simulink model "flexpes_phctrlr_backup_jun3_2022"  (R2020a)
settings: Solver=VariableStepAuto  StartTime=0.0  StopTime=10.0  RelTol=1e-3
undefined symbols (not defined in the file): debouncer_cycles, F_lock_thr, FPGA_CLK, FPGA_Ts, IIR_C_X, IIR_C_X1, IIR_C_Y1, max_unwrap_periods, PFD_CLK, PFD_Ts, PH_lock_thr, PHCTRLR_CLK, PHCTRLR_Ts, TDC_cnt_per_period, unwrap_res_period_thr, unwrap_res_thr, wrap_detect_thr
libraries: xbsIndex_r4 x277
(part 2 of 2)

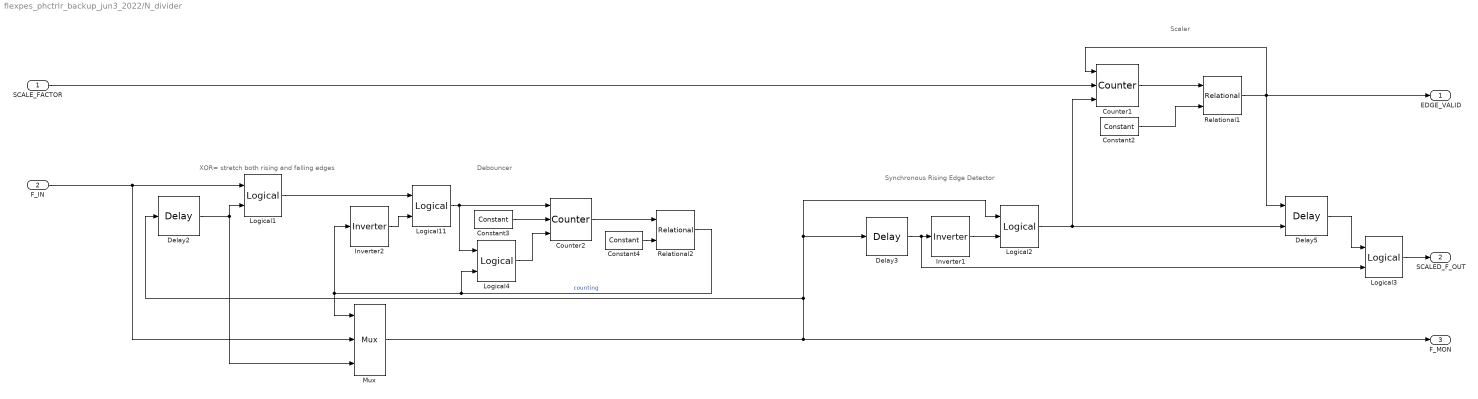
== system flexpes_phctrlr_backup_jun3_2022/N_divider ==
  note: XOR= stretch both rising and falling edges
  note: Debouncer
  note: Scaler
  note: Synchronous Rising Edge Detector
  SCALE_FACTOR : Inport
  F_IN : Inport  Port=2
  Constant2 : xbsIndex_r4/Constant  const=1.0  gui_display_data_type=Fixed-point  arith_type=Unsigned  n_bits=10  bin_pt=0  preci_type=Single  exp_width=8  frac_width=24  explicit_period=off  period=1  equ=P=C  opselect=C  inp2=PCIN>>17  opr=+  inp1=P  carry=CIN  dbl_ovrd=off  block_type=constant
  Constant3 : xbsIndex_r4/Constant  const=debouncer_cycles  gui_display_data_type=Fixed-point  arith_type=Unsigned  n_bits=7  bin_pt=0  preci_type=Single  exp_width=8  frac_width=24  explicit_period=off  period=1  equ=P=C  opselect=C  inp2=PCIN>>17  opr=+  inp1=P  carry=CIN  dbl_ovrd=off  block_type=constant
  Constant4 : xbsIndex_r4/Constant  const=1  gui_display_data_type=Fixed-point  arith_type=Unsigned  n_bits=7  bin_pt=0  preci_type=Single  exp_width=8  frac_width=24  explicit_period=off  period=1  equ=P=C  opselect=C  inp2=PCIN>>17  opr=+  inp1=P  carry=CIN  dbl_ovrd=off  block_type=constant
  Counter1 : xbsIndex_r4/Counter  cnt_type=Free Running  cnt_to=2  operation=Down  start_count=1  cnt_by_val=1  arith_type=Unsigned  n_bits=10  bin_pt=0  load_pin=on  rst=off  en=on  explicit_period=on  period=FPGA_Ts  use_behavioral_HDL=off  implementation=Fabric  dbl_ovrd=off  block_type=counter
  Counter2 : xbsIndex_r4/Counter  cnt_type=Free Running  cnt_to=2  operation=Down  start_count=1  cnt_by_val=1  arith_type=Unsigned  n_bits=7  bin_pt=0  load_pin=on  rst=off  en=on  explicit_period=on  period=FPGA_Ts  use_behavioral_HDL=off  implementation=Fabric  dbl_ovrd=off  block_type=counter
  Delay2 : xbsIndex_r4/Delay  rst=off  infoeditControl=Selection of Reset will increase slice count due to use of real FFs and instead of SRLs  en=off  latency=1  reg_retiming=off  dbl_ovrd=off  block_type=delay
  Delay3 : xbsIndex_r4/Delay  rst=off  infoeditControl=Selection of Reset will increase slice count due to use of real FFs and instead of SRLs  en=off  latency=1  reg_retiming=off  dbl_ovrd=off  block_type=delay
  Delay5 : xbsIndex_r4/Delay  rst=off  infoeditControl=Selection of Reset will increase slice count due to use of real FFs and instead of SRLs  en=on  latency=1  reg_retiming=off  dbl_ovrd=off  block_type=delay
  Inverter1 : xbsIndex_r4/Inverter  en=off  latency=0  dbl_ovrd=off  block_type=inv
  Inverter2 : xbsIndex_r4/Inverter  en=off  latency=0  dbl_ovrd=off  block_type=inv
  Logical1 : xbsIndex_r4/Logical  logical_function=XOR  inputs=2  en=off  latency=0  precision=Full  arith_type=Unsigned  n_bits=16  bin_pt=0  align_bp=on  dbl_ovrd=off  block_type=logical
  Logical11 : xbsIndex_r4/Logical  logical_function=AND  inputs=2  en=off  latency=0  precision=Full  arith_type=Unsigned  n_bits=16  bin_pt=0  align_bp=on  dbl_ovrd=off  block_type=logical
  Logical2 : xbsIndex_r4/Logical  logical_function=AND  inputs=2  en=off  latency=0  precision=Full  arith_type=Unsigned  n_bits=16  bin_pt=0  align_bp=on  dbl_ovrd=off  block_type=logical
  Logical3 : xbsIndex_r4/Logical  logical_function=AND  inputs=2  en=off  latency=0  precision=Full  arith_type=Unsigned  n_bits=16  bin_pt=0  align_bp=on  dbl_ovrd=off  block_type=logical
  Logical4 : xbsIndex_r4/Logical  logical_function=OR  inputs=2  en=off  latency=0  precision=Full  arith_type=Unsigned  n_bits=16  bin_pt=0  align_bp=on  dbl_ovrd=off  block_type=logical
  Mux : xbsIndex_r4/Mux  inputs=2  en=off  latency=0  precision=Full  arith_type=Unsigned  n_bits=16  bin_pt=14  quantization=Truncate  overflow=Wrap  dbl_ovrd=off  block_type=mux
  Relational1 : xbsIndex_r4/Relational  mode=a=b  op_type=Bool  en=off  latency=0  dbl_ovrd=off  block_type=relational
  Relational2 : xbsIndex_r4/Relational  mode=a!=b  op_type=Bool  en=off  latency=0  dbl_ovrd=off  block_type=relational
  EDGE_VALID : Outport
  SCALED_F_OUT : Outport  Port=2
  F_MON : Outport  Port=3
  wires:
  Delay2/1 -> Logical1/2, Mux/3
  Logical2/1 -> Delay5/2, Counter1/3
  Constant4/1 -> Relational2/2
  Inverter2/1 -> Logical11/2
  Counter2/1 -> Relational2/1
  Constant3/1 -> Counter2/2
  Relational2/1 -> Mux/1, Inverter2/1, Logical4/2  "counting"
  Delay5/1 -> Logical3/1
  Delay3/1 -> Inverter1/1, Logical3/2
  F_IN/1 -> Logical1/1, Mux/2
  Counter1/1 -> Relational1/1
  Inverter1/1 -> Logical2/2
  Constant2/1 -> Relational1/2
  SCALE_FACTOR/1 -> Counter1/2
  Logical11/1 -> Logical4/1, Counter2/1
  Logical3/1 -> SCALED_F_OUT/1
  Logical4/1 -> Counter2/3
  Logical1/1 -> Logical11/1
  Relational1/1 -> EDGE_VALID/1, Delay5/1, Counter1/1
  Mux/1 -> F_MON/1, Delay2/1, Logical2/1, Delay3/1

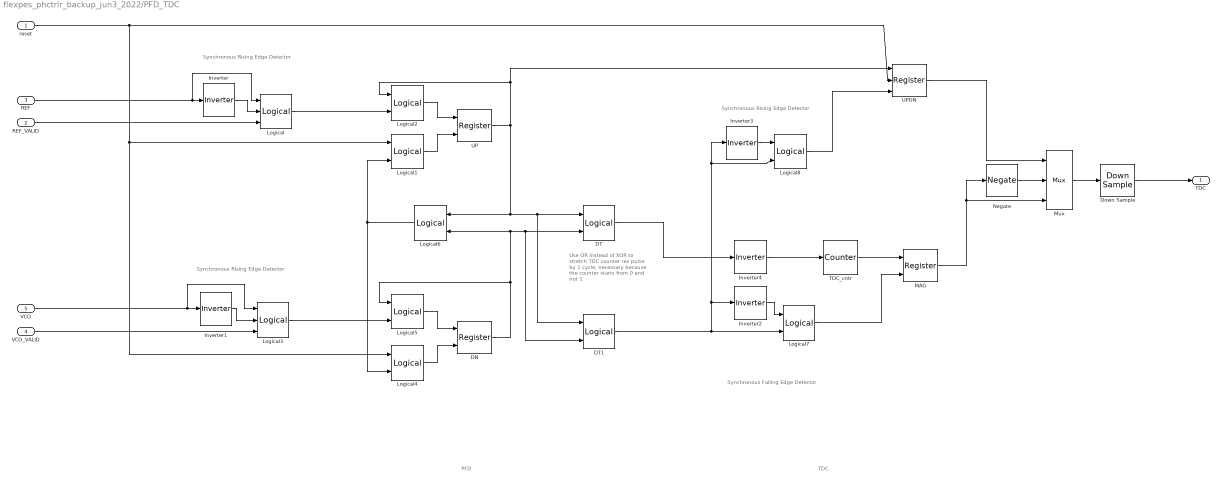
== system flexpes_phctrlr_backup_jun3_2022/PFD_TDC ==
  note: Synchronous Rising Edge Detector
  note: Synchronous Rising Edge Detector
  note: Synchronous Rising Edge Detector
  note: Synchronous Falling Edge Detector
  note: PFD
  note: TDC
  note: Use OR instead of XOR to
      | stretch TDC counter res
      | pulse by 1 cycle, necessary
      | because the counter starts
      | from 0 and not 1
  reset : Inport  SampleTime=FPGA_Ts
  REF_VALID : Inport  Port=2  SampleTime=FPGA_Ts
  REF : Inport  Port=3  SampleTime=FPGA_Ts
  VCO_VALID : Inport  Port=4  SampleTime=FPGA_Ts
  VCO : Inport  Port=5  SampleTime=FPGA_Ts
  DN : xbsIndex_r4/Register  init=0  rst=on  en=off  dbl_ovrd=off  block_type=register
  DT : xbsIndex_r4/Logical  logical_function=OR  inputs=2  en=off  latency=0  precision=Full  arith_type=Unsigned  n_bits=16  bin_pt=0  align_bp=on  dbl_ovrd=off  block_type=logical
  DT1 : xbsIndex_r4/Logical  logical_function=XOR  inputs=2  en=off  latency=0  precision=Full  arith_type=Unsigned  n_bits=16  bin_pt=0  align_bp=on  dbl_ovrd=off  block_type=logical
  Down Sample : xbsIndex_r4/Down Sample  sample_ratio=FPGA_CLK/PFD_CLK  sample_phase="Last Value of Frame  (most efficient)"  en=off  rst=off  latency=1  dbl_ovrd=off  block_type=dsamp
  Inverter{,1..3} (4 alike) : xbsIndex_r4/Inverter  en=off  latency=1  dbl_ovrd=off  block_type=inv
  Inverter4 : xbsIndex_r4/Inverter  en=off  latency=0  dbl_ovrd=off  block_type=inv
  Logical : xbsIndex_r4/Logical  logical_function=AND  inputs=3  en=off  latency=0  precision=Full  arith_type=Unsigned  n_bits=16  bin_pt=0  align_bp=on  dbl_ovrd=off  block_type=logical
  Logical{1..2,4..5} (4 alike) : xbsIndex_r4/Logical  logical_function=OR  inputs=2  en=off  latency=0  precision=Full  arith_type=Unsigned  n_bits=16  bin_pt=0  align_bp=on  dbl_ovrd=off  block_type=logical
  Logical3 : xbsIndex_r4/Logical  logical_function=AND  inputs=3  en=off  latency=0  precision=Full  arith_type=Unsigned  n_bits=16  bin_pt=0  align_bp=on  dbl_ovrd=off  block_type=logical
  Logical6 : xbsIndex_r4/Logical  logical_function=AND  inputs=2  en=off  latency=1  precision=Full  arith_type=Unsigned  n_bits=16  bin_pt=0  align_bp=on  dbl_ovrd=off  block_type=logical
  Logical7 : xbsIndex_r4/Logical  logical_function=NOR  inputs=2  en=off  latency=0  precision=Full  arith_type=Unsigned  n_bits=16  bin_pt=0  align_bp=on  dbl_ovrd=off  block_type=logical
  Logical8 : xbsIndex_r4/Logical  logical_function=AND  inputs=2  en=off  latency=0  precision=Full  arith_type=Unsigned  n_bits=16  bin_pt=0  align_bp=on  dbl_ovrd=off  block_type=logical
  MAG : xbsIndex_r4/Register  init=0  rst=off  en=on  dbl_ovrd=off  block_type=register
  Mux : xbsIndex_r4/Mux  inputs=2  en=off  latency=1  precision=Full  arith_type=Unsigned  n_bits=16  bin_pt=14  quantization=Truncate  overflow=Wrap  dbl_ovrd=off  block_type=mux
  Negate : xbsIndex_r4/Negate  precision=User Defined  arith_type="Signed  (2's comp)"  n_bits=17  bin_pt=0  quantization=Truncate  overflow=Wrap  en=off  latency=0  dbl_ovrd=off  block_type=negate
  TDC_cntr : xbsIndex_r4/Counter  cnt_type=Free Running  cnt_to=Inf  operation=Up  start_count=0  cnt_by_val=1  arith_type="Signed  (2's comp)"  n_bits=17  bin_pt=0  load_pin=off  rst=on  en=off  explicit_period=on  period=FPGA_Ts  use_behavioral_HDL=off  implementation=DSP48  dbl_ovrd=off  block_type=counter
  UP : xbsIndex_r4/Register  init=0  rst=on  en=off  dbl_ovrd=off  block_type=register
  UPDN : xbsIndex_r4/Register  init=0  rst=on  en=on  dbl_ovrd=off  block_type=register
  TDC : Outport  SampleTime=PFD_Ts
  wires:
  Logical3/1 -> Logical5/2
  VCO/1 -> Logical3/1, Inverter1/1
  reset/1 -> Logical4/1, Logical1/1, UPDN/2
  Logical5/1 -> DN/1
  Logical2/1 -> UP/1
  DN/1 -> Logical5/1, Logical6/2, DT1/2, DT/2
  REF/1 -> Logical/1, Inverter/1
  DT/1 -> Inverter4/1
  Logical4/1 -> DN/2
  MAG/1 -> Negate/1, Mux/3
  Down Sample/1 -> TDC/1
  Inverter3/1 -> Logical8/1
  Logical8/1 -> UPDN/3
  UP/1 -> UPDN/1, Logical2/1, DT1/1, DT/1, Logical6/1
  Logical6/1 -> Logical1/2, Logical4/2
  Logical1/1 -> UP/2
  UPDN/1 -> Mux/1
  Mux/1 -> Down Sample/1
  Logical/1 -> Logical2/2
  Negate/1 -> Mux/2
  Logical7/1 -> MAG/2
  Inverter2/1 -> Logical7/1
  TDC_cntr/1 -> MAG/1
  Inverter4/1 -> TDC_cntr/1
  DT1/1 -> Logical8/2, Inverter3/1, Inverter2/1, Logical7/2
  REF_VALID/1 -> Logical/3
  Inverter1/1 -> Logical3/2
  VCO_VALID/1 -> Logical3/3
  Inverter/1 -> Logical/2

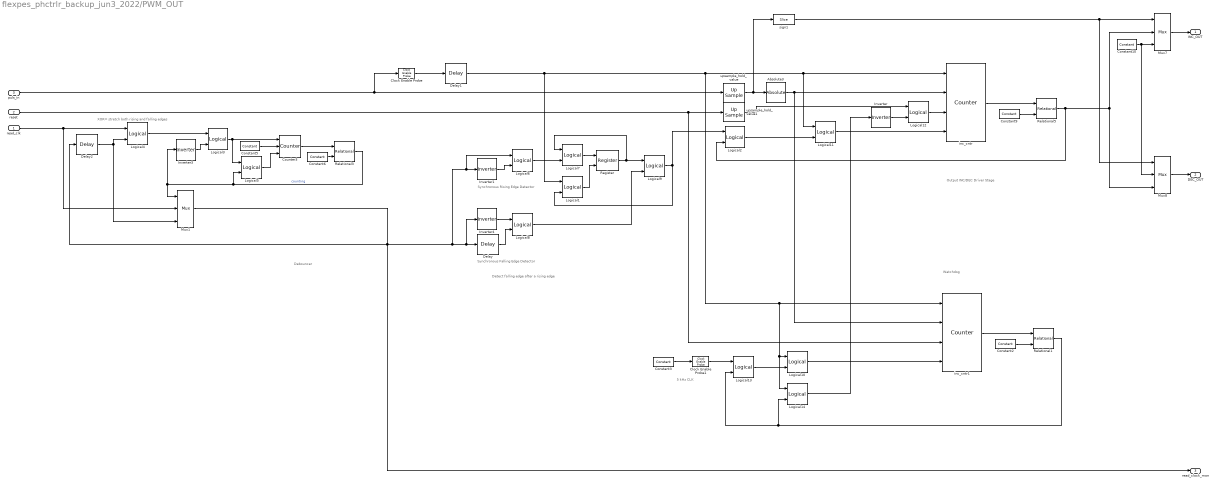
== system flexpes_phctrlr_backup_jun3_2022/PWM_OUT ==
  note: Output INC/DEC Driver Stage
  note: XOR= stretch both rising and falling edges
  note: Synchronous Rising Edge Detector
  note: Detect falling edge after a rising edge
  note: Debouncer
  note: Watchdog
  note: Synchronous Falling Edge Detector
  note: 5 kHz CLK
  read_clk : Inport
  reset : Inport  Port=2
  puls_in : Inport  Port=3
  Absolute3 : xbsIndex_r4/Absolute  precision=User Defined  arith_type="Signed  (2's comp)"  n_bits=22  bin_pt=0  quantization=Truncate  overflow=Wrap  en=off  latency=0  dbl_ovrd=off  block_type=abs
  Clock Enable Probe : xbsIndex_r4/Clock Enable Probe  inherit_constraints=on  block_type=ceprobe
      settings: infoedit="Clock enable extractor.  Produces a Boolean output that mirrors the hardware clock enable associated with the input sample rate.<br><br>Hardware notes: in hardware this block costs nothing."
  Clock Enable Probe1 : xbsIndex_r4/Clock Enable Probe  inherit_constraints=on  block_type=ceprobe
      settings: infoedit="Clock enable extractor.  Produces a Boolean output that mirrors the hardware clock enable associated with the input sample rate.<br><br>Hardware notes: in hardware this block costs nothing."
  Constant10 : xbsIndex_r4/Constant  const=0  gui_display_data_type=Boolean  arith_type=Boolean  n_bits=22  bin_pt=0  preci_type=Single  exp_width=8  frac_width=24  explicit_period=off  period=1  equ=P=C  opselect=C  inp2=PCIN>>17  opr=+  inp1=P  carry=CIN  dbl_ovrd=off  block_type=constant
  Constant2 : xbsIndex_r4/Constant  const=0  gui_display_data_type=Fixed-point  arith_type=Signed (2's comp)  n_bits=22  bin_pt=0  preci_type=Single  exp_width=8  frac_width=24  explicit_period=off  period=1  equ=P=C  opselect=C  inp2=PCIN>>17  opr=+  inp1=P  carry=CIN  dbl_ovrd=off  block_type=constant
  Constant3 : xbsIndex_r4/Constant  const=1  gui_display_data_type=Boolean  arith_type=Boolean  n_bits=7  bin_pt=0  preci_type=Single  exp_width=8  frac_width=24  explicit_period=on  period=PWM_Ts  equ=P=C  opselect=C  inp2=PCIN>>17  opr=+  inp1=P  carry=CIN  dbl_ovrd=off  block_type=constant
  Constant5 : xbsIndex_r4/Constant  const=debouncer_cycles  gui_display_data_type=Fixed-point  arith_type=Unsigned  n_bits=7  bin_pt=0  preci_type=Single  exp_width=8  frac_width=24  explicit_period=off  period=1  equ=P=C  opselect=C  inp2=PCIN>>17  opr=+  inp1=P  carry=CIN  dbl_ovrd=off  block_type=constant
  Constant6 : xbsIndex_r4/Constant  const=1  gui_display_data_type=Fixed-point  arith_type=Unsigned  n_bits=7  bin_pt=0  preci_type=Single  exp_width=8  frac_width=24  explicit_period=off  period=1  equ=P=C  opselect=C  inp2=PCIN>>17  opr=+  inp1=P  carry=CIN  dbl_ovrd=off  block_type=constant
  Constant9 : xbsIndex_r4/Constant  const=0  gui_display_data_type=Fixed-point  arith_type=Signed (2's comp)  n_bits=22  bin_pt=0  preci_type=Single  exp_width=8  frac_width=24  explicit_period=off  period=1  equ=P=C  opselect=C  inp2=PCIN>>17  opr=+  inp1=P  carry=CIN  dbl_ovrd=off  block_type=constant
  Counter3 : xbsIndex_r4/Counter  cnt_type=Free Running  cnt_to=2  operation=Down  start_count=1  cnt_by_val=1  arith_type=Unsigned  n_bits=7  bin_pt=0  load_pin=on  rst=off  en=on  explicit_period=on  period=FPGA_Ts  use_behavioral_HDL=off  implementation=Fabric  dbl_ovrd=off  block_type=counter
  Delay : xbsIndex_r4/Delay  rst=off  infoeditControl=Selection of Reset will increase slice count due to use of real FFs and instead of SRLs  en=off  latency=1  reg_retiming=off  dbl_ovrd=off  block_type=delay
  Delay1 : xbsIndex_r4/Delay  rst=off  infoeditControl=Selection of Reset will increase slice count due to use of real FFs and instead of SRLs  en=off  latency=1  reg_retiming=off  dbl_ovrd=off  block_type=delay
  Delay2 : xbsIndex_r4/Delay  rst=off  infoeditControl=Selection of Reset will increase slice count due to use of real FFs and instead of SRLs  en=off  latency=1  reg_retiming=off  dbl_ovrd=off  block_type=delay
  Inverter : xbsIndex_r4/Inverter  en=off  latency=0  dbl_ovrd=off  block_type=inv
  Inverter1 : xbsIndex_r4/Inverter  en=off  latency=1  dbl_ovrd=off  block_type=inv
  Inverter3 : xbsIndex_r4/Inverter  en=off  latency=0  dbl_ovrd=off  block_type=inv
  Inverter4 : xbsIndex_r4/Inverter  en=off  latency=0  dbl_ovrd=off  block_type=inv
  Logical{1,5,7,10..12,14} (7 alike) : xbsIndex_r4/Logical  logical_function=OR  inputs=2  en=off  latency=0  precision=Full  arith_type=Unsigned  n_bits=16  bin_pt=0  align_bp=on  dbl_ovrd=off  block_type=logical
  Logical{2..3,6,8..9,13} (6 alike) : xbsIndex_r4/Logical  logical_function=AND  inputs=2  en=off  latency=0  precision=Full  arith_type=Unsigned  n_bits=16  bin_pt=0  align_bp=on  dbl_ovrd=off  block_type=logical
  Logical4 : xbsIndex_r4/Logical  logical_function=XOR  inputs=2  en=off  latency=0  precision=Full  arith_type=Unsigned  n_bits=16  bin_pt=0  align_bp=on  dbl_ovrd=off  block_type=logical
  Mux1 : xbsIndex_r4/Mux  inputs=2  en=off  latency=0  precision=Full  arith_type=Unsigned  n_bits=16  bin_pt=14  quantization=Truncate  overflow=Wrap  dbl_ovrd=off  block_type=mux
  Mux7 : xbsIndex_r4/Mux  inputs=2  en=off  latency=0  precision=Full  arith_type=Unsigned  n_bits=16  bin_pt=14  quantization=Truncate  overflow=Wrap  dbl_ovrd=off  block_type=mux
  Mux8 : xbsIndex_r4/Mux  inputs=2  en=off  latency=0  precision=Full  arith_type=Unsigned  n_bits=16  bin_pt=14  quantization=Truncate  overflow=Wrap  dbl_ovrd=off  block_type=mux
  Register : xbsIndex_r4/Register  init=0  rst=on  en=off  dbl_ovrd=off  block_type=register
  Relational1 : xbsIndex_r4/Relational  mode=a!=b  op_type=Bool  en=off  latency=0  dbl_ovrd=off  block_type=relational
  Relational3 : xbsIndex_r4/Relational  mode=a!=b  op_type=Bool  en=off  latency=0  dbl_ovrd=off  block_type=relational
  Relational5 : xbsIndex_r4/Relational  mode=a!=b  op_type=Bool  en=off  latency=0  dbl_ovrd=off  block_type=relational
  inc_cntr : xbsIndex_r4/Counter  cnt_type=Free Running  cnt_to=0  operation=Down  start_count=0  cnt_by_val=1  arith_type="Signed  (2's comp)"  n_bits=22  bin_pt=0  load_pin=on  rst=on  en=on  explicit_period=on  period=FPGA_Ts  use_behavioral_HDL=off  implementation=DSP48  dbl_ovrd=off  block_type=counter
  inc_cntr1 : xbsIndex_r4/Counter  cnt_type=Free Running  cnt_to=0  operation=Down  start_count=0  cnt_by_val=1  arith_type="Signed  (2's comp)"  n_bits=22  bin_pt=0  load_pin=on  rst=on  en=on  explicit_period=on  period=FPGA_Ts  use_behavioral_HDL=off  implementation=DSP48  dbl_ovrd=off  block_type=counter
  sign1 : xbsIndex_r4/Slice  nbits=1  boolean_output=on  mode=Upper Bit Location + Width  bit1=0  base1=MSB of Input  bit0=0  base0=LSB of Input  dbl_ovrd=off  block_type=slice
  upsample_hold_value : xbsIndex_r4/Up Sample  sample_ratio=FPGA_CLK/PHCTRLR_CLK  copy_samples=on  en=off  latency=0  dbl_ovrd=off  block_type=usamp
  upsample_hold_value1 : xbsIndex_r4/Up Sample  sample_ratio=FPGA_CLK/PHCTRLR_CLK  copy_samples=on  en=off  latency=0  dbl_ovrd=off  block_type=usamp
  INC_OUT : Outport
  DEC_OUT : Outport  Port=2
  read_clock_mon : Outport  Port=3
  wires:
  Logical14/1 -> Inverter/1
  Logical10/1 -> inc_cntr1/4
  Clock Enable Probe/1 -> Delay1/1
  Delay1/1 -> Logical1/1, Logical14/1, Logical10/1, inc_cntr1/1, inc_cntr/1, Logical11/1
  Inverter/1 -> Logical12/2
  Clock Enable Probe1/1 -> Logical13/1
  inc_cntr1/1 -> Relational1/1
  Logical7/1 -> Register/1
  upsample_hold_value1/1 -> Logical12/1
  Logical6/1 -> Logical7/2
  Logical11/1 -> inc_cntr/4
  Counter3/1 -> Relational3/1
  Logical8/1 -> Logical9/2
  puls_in/1 -> upsample_hold_value/1, Clock Enable Probe/1
  Constant2/1 -> Relational1/2
  Mux7/1 -> INC_OUT/1
  Constant5/1 -> Counter3/2
  reset/1 -> inc_cntr1/3, upsample_hold_value1/1
  Logical12/1 -> inc_cntr/3
  Constant6/1 -> Relational3/2
  Delay/1 -> Logical8/2
  Inverter3/1 -> Logical3/2
  Relational3/1 -> Mux1/1, Inverter3/1, Logical5/2  "counting"
  Relational5/1 -> Logical2/2, Mux8/3, Mux7/2
  Logical5/1 -> Counter3/3
  Register/1 -> Logical9/1, Logical7/1
  Inverter1/1 -> Logical6/2
  read_clk/1 -> Logical4/1, Mux1/2
  Logical9/1 -> Logical1/2, Logical2/1
  Logical4/1 -> Logical3/1
  Delay2/1 -> Mux1/3, Logical4/2
  Logical2/1 -> Logical11/2
  Absolute3/1 -> inc_cntr/2, inc_cntr1/2
  sign1/1 -> Mux8/1, Mux7/1
  Constant9/1 -> Relational5/2
  Logical13/1 -> Logical10/2
  Inverter4/1 -> Logical8/1
  Mux1/1 -> read_clock_mon/1, Delay2/1, Logical6/1, Inverter1/1, Inverter4/1, Delay/1
  Mux8/1 -> DEC_OUT/1
  Constant10/1 -> Mux8/2, Mux7/3
  Relational1/1 -> Logical14/2, Logical13/2
  Constant3/1 -> Clock Enable Probe1/1
  Logical3/1 -> Logical5/1, Counter3/1
  Logical1/1 -> Register/2
  inc_cntr/1 -> Relational5/1
  upsample_hold_value/1 -> sign1/1, Absolute3/1

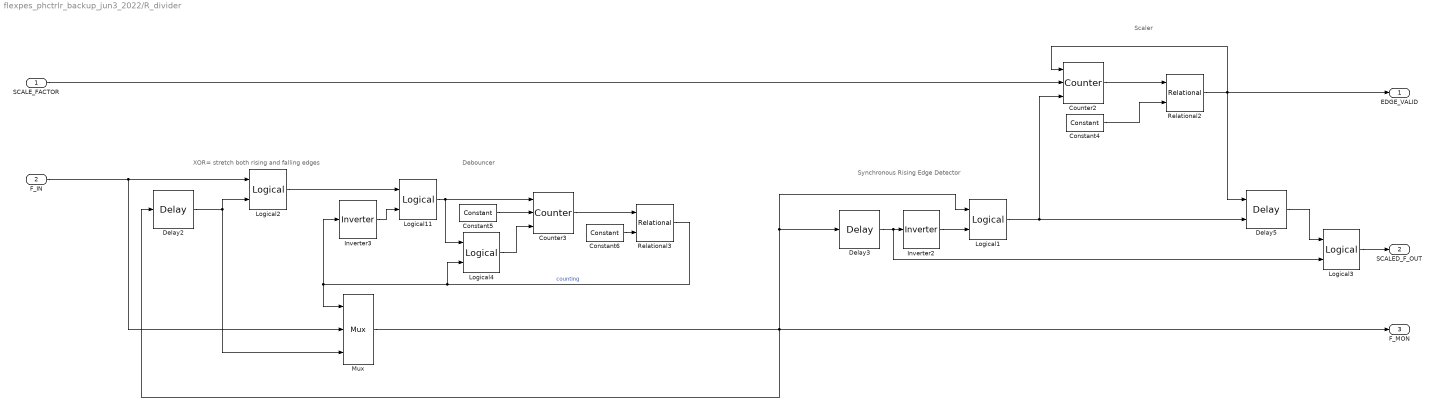
== system flexpes_phctrlr_backup_jun3_2022/R_divider ==
  note: XOR= stretch both rising and falling edges
  note: Debouncer
  note: Scaler
  note: Synchronous Rising Edge Detector
  SCALE_FACTOR : Inport
  F_IN : Inport  Port=2
  Constant4 : xbsIndex_r4/Constant  const=1.0  gui_display_data_type=Fixed-point  arith_type=Unsigned  n_bits=10  bin_pt=0  preci_type=Single  exp_width=8  frac_width=24  explicit_period=off  period=1  equ=P=C  opselect=C  inp2=PCIN>>17  opr=+  inp1=P  carry=CIN  dbl_ovrd=off  block_type=constant
  Constant5 : xbsIndex_r4/Constant  const=debouncer_cycles  gui_display_data_type=Fixed-point  arith_type=Unsigned  n_bits=7  bin_pt=0  preci_type=Single  exp_width=8  frac_width=24  explicit_period=off  period=1  equ=P=C  opselect=C  inp2=PCIN>>17  opr=+  inp1=P  carry=CIN  dbl_ovrd=off  block_type=constant
  Constant6 : xbsIndex_r4/Constant  const=1  gui_display_data_type=Fixed-point  arith_type=Unsigned  n_bits=7  bin_pt=0  preci_type=Single  exp_width=8  frac_width=24  explicit_period=off  period=1  equ=P=C  opselect=C  inp2=PCIN>>17  opr=+  inp1=P  carry=CIN  dbl_ovrd=off  block_type=constant
  Counter2 : xbsIndex_r4/Counter  cnt_type=Free Running  cnt_to=2  operation=Down  start_count=1  cnt_by_val=1  arith_type=Unsigned  n_bits=10  bin_pt=0  load_pin=on  rst=off  en=on  explicit_period=on  period=FPGA_Ts  use_behavioral_HDL=off  implementation=Fabric  dbl_ovrd=off  block_type=counter
  Counter3 : xbsIndex_r4/Counter  cnt_type=Free Running  cnt_to=2  operation=Down  start_count=1  cnt_by_val=1  arith_type=Unsigned  n_bits=7  bin_pt=0  load_pin=on  rst=off  en=on  explicit_period=on  period=FPGA_Ts  use_behavioral_HDL=off  implementation=Fabric  dbl_ovrd=off  block_type=counter
  Delay2 : xbsIndex_r4/Delay  rst=off  infoeditControl=Selection of Reset will increase slice count due to use of real FFs and instead of SRLs  en=off  latency=1  reg_retiming=off  dbl_ovrd=off  block_type=delay
  Delay3 : xbsIndex_r4/Delay  rst=off  infoeditControl=Selection of Reset will increase slice count due to use of real FFs and instead of SRLs  en=off  latency=1  reg_retiming=off  dbl_ovrd=off  block_type=delay
  Delay5 : xbsIndex_r4/Delay  rst=off  infoeditControl=Selection of Reset will increase slice count due to use of real FFs and instead of SRLs  en=on  latency=1  reg_retiming=off  dbl_ovrd=off  block_type=delay
  Inverter2 : xbsIndex_r4/Inverter  en=off  latency=0  dbl_ovrd=off  block_type=inv
  Inverter3 : xbsIndex_r4/Inverter  en=off  latency=0  dbl_ovrd=off  block_type=inv
  Logical1 : xbsIndex_r4/Logical  logical_function=AND  inputs=2  en=off  latency=0  precision=Full  arith_type=Unsigned  n_bits=16  bin_pt=0  align_bp=on  dbl_ovrd=off  block_type=logical
  Logical11 : xbsIndex_r4/Logical  logical_function=AND  inputs=2  en=off  latency=0  precision=Full  arith_type=Unsigned  n_bits=16  bin_pt=0  align_bp=on  dbl_ovrd=off  block_type=logical
  Logical2 : xbsIndex_r4/Logical  logical_function=XOR  inputs=2  en=off  latency=0  precision=Full  arith_type=Unsigned  n_bits=16  bin_pt=0  align_bp=on  dbl_ovrd=off  block_type=logical
  Logical3 : xbsIndex_r4/Logical  logical_function=AND  inputs=2  en=off  latency=0  precision=Full  arith_type=Unsigned  n_bits=16  bin_pt=0  align_bp=on  dbl_ovrd=off  block_type=logical
  Logical4 : xbsIndex_r4/Logical  logical_function=OR  inputs=2  en=off  latency=0  precision=Full  arith_type=Unsigned  n_bits=16  bin_pt=0  align_bp=on  dbl_ovrd=off  block_type=logical
  Mux : xbsIndex_r4/Mux  inputs=2  en=off  latency=0  precision=Full  arith_type=Unsigned  n_bits=16  bin_pt=14  quantization=Truncate  overflow=Wrap  dbl_ovrd=off  block_type=mux
  Relational2 : xbsIndex_r4/Relational  mode=a=b  op_type=Bool  en=off  latency=0  dbl_ovrd=off  block_type=relational
  Relational3 : xbsIndex_r4/Relational  mode=a!=b  op_type=Bool  en=off  latency=0  dbl_ovrd=off  block_type=relational
  EDGE_VALID : Outport
  SCALED_F_OUT : Outport  Port=2
  F_MON : Outport  Port=3
  wires:
  Logical1/1 -> Counter2/3, Delay5/2
  Constant6/1 -> Relational3/2
  Inverter3/1 -> Logical11/2
  Counter3/1 -> Relational3/1
  Constant5/1 -> Counter3/2
  Relational3/1 -> Mux/1, Inverter3/1, Logical4/2  "counting"
  Delay5/1 -> Logical3/1
  Delay3/1 -> Inverter2/1, Logical3/2
  F_IN/1 -> Logical2/1, Mux/2
  Counter2/1 -> Relational2/1
  Inverter2/1 -> Logical1/2
  Constant4/1 -> Relational2/2
  SCALE_FACTOR/1 -> Counter2/2
  Logical11/1 -> Logical4/1, Counter3/1
  Logical3/1 -> SCALED_F_OUT/1
  Logical4/1 -> Counter3/3
  Logical2/1 -> Logical11/1
  Delay2/1 -> Mux/3, Logical2/2
  Relational2/1 -> EDGE_VALID/1, Delay5/1, Counter2/1
  Mux/1 -> F_MON/1, Delay2/1, Logical1/1, Delay3/1

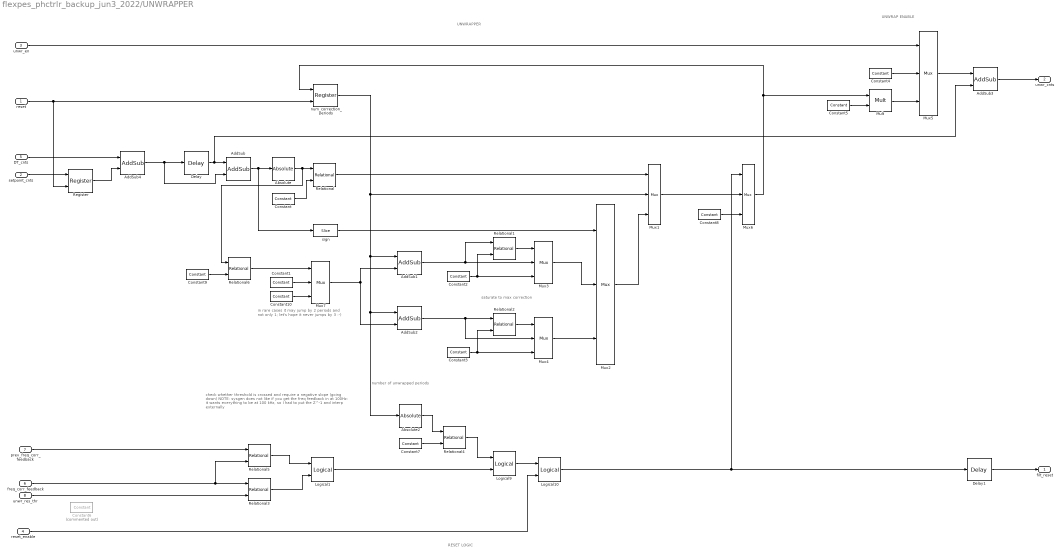
== system flexpes_phctrlr_backup_jun3_2022/UNWRAPPER ==
  note: UNWRAPPER
  note: saturate to max correction
  note: RESET LOGIC
  note: UNWRAP ENABLE
  note: check whether threshold is crossed and require
      | a negative slope (going down)
      | NOTE: sysgen does not like if you get the freq feedback in
      | at 100Hz: it wants everything to be at 100 kHz, so I had to
      | put the Z^-1 and interp externally
  note: number of unwrapped periods
  note: in rare cases it may jump by 2 periods and not only 1; let's hope it never jumps by 3 :-)
  reset : Inport
  setpoint_cnts : Inport  Port=2
  unwr_en : Inport  Port=3
  reset_enable : Inport  Port=4
  DT_cnts : Inport  Port=5
  freq_corr_feedback : Inport  Port=6
  prev_freq_corr_feedback : Inport  Port=7
  unwr_res_thr : Inport  Port=8
  Absolute : xbsIndex_r4/Absolute  precision=User Defined  arith_type="Signed  (2's comp)"  n_bits=17  bin_pt=0  quantization=Truncate  overflow=Saturate  en=off  latency=0  dbl_ovrd=off  block_type=abs
  Absolute2 : xbsIndex_r4/Absolute  precision=User Defined  arith_type="Signed  (2's comp)"  n_bits=17  bin_pt=0  quantization=Truncate  overflow=Saturate  en=off  latency=0  dbl_ovrd=off  block_type=abs
  AddSub : xbsIndex_r4/AddSub  mode=Subtraction  use_carryin=off  use_carryout=off  en=off  latency=1  precision=User Defined  arith_type="Signed  (2's comp)"  n_bits=17  bin_pt=0  quantization=Truncate  overflow=Saturate  use_behavioral_HDL=off  hw_selection=Fabric  pipelined=off  dbl_ovrd=off  block_type=addsub
  AddSub1 : xbsIndex_r4/AddSub  mode=Addition  use_carryin=off  use_carryout=off  en=off  latency=0  precision=User Defined  arith_type="Signed  (2's comp)"  n_bits=7  bin_pt=0  quantization=Truncate  overflow=Saturate  use_behavioral_HDL=off  hw_selection=Fabric  pipelined=off  dbl_ovrd=off  block_type=addsub
  AddSub2 : xbsIndex_r4/AddSub  mode=Subtraction  use_carryin=off  use_carryout=off  en=off  latency=0  precision=User Defined  arith_type="Signed  (2's comp)"  n_bits=7  bin_pt=0  quantization=Truncate  overflow=Saturate  use_behavioral_HDL=off  hw_selection=Fabric  pipelined=off  dbl_ovrd=off  block_type=addsub
  AddSub3 : xbsIndex_r4/AddSub  mode=Addition  use_carryin=off  use_carryout=off  en=off  latency=0  precision=User Defined  arith_type="Signed  (2's comp)"  n_bits=17  bin_pt=0  quantization="Round  (unbiased: +/- Inf)"  overflow=Saturate  use_behavioral_HDL=off  hw_selection=Fabric  pipelined=off  dbl_ovrd=off  block_type=addsub
  AddSub4 : xbsIndex_r4/AddSub  mode=Subtraction  use_carryin=off  use_carryout=off  en=off  latency=1  precision=User Defined  arith_type="Signed  (2's comp)"  n_bits=17  bin_pt=0  quantization="Round  (unbiased: +/- Inf)"  overflow=Saturate  use_behavioral_HDL=off  hw_selection=Fabric  pipelined=off  dbl_ovrd=off  block_type=addsub
  Constant : xbsIndex_r4/Constant  const=wrap_detect_thr  gui_display_data_type=Fixed-point  arith_type=Signed (2's comp)  n_bits=17  bin_pt=0  preci_type=Single  exp_width=8  frac_width=24  explicit_period=off  period=1  equ=P=C  opselect=C  inp2=PCIN>>17  opr=+  inp1=P  carry=CIN  dbl_ovrd=off  block_type=constant
  Constant1 : xbsIndex_r4/Constant  const=1  gui_display_data_type=Fixed-point  arith_type=Signed (2's comp)  n_bits=7  bin_pt=0  preci_type=Single  exp_width=8  frac_width=24  explicit_period=off  period=1  equ=P=C  opselect=C  inp2=PCIN>>17  opr=+  inp1=P  carry=CIN  dbl_ovrd=off  block_type=constant
  Constant10 : xbsIndex_r4/Constant  const=2  gui_display_data_type=Fixed-point  arith_type=Signed (2's comp)  n_bits=7  bin_pt=0  preci_type=Single  exp_width=8  frac_width=24  explicit_period=off  period=1  equ=P=C  opselect=C  inp2=PCIN>>17  opr=+  inp1=P  carry=CIN  dbl_ovrd=off  block_type=constant
  Constant2 : xbsIndex_r4/Constant  const=max_unwrap_periods  gui_display_data_type=Fixed-point  arith_type=Signed (2's comp)  n_bits=7  bin_pt=0  preci_type=Single  exp_width=8  frac_width=24  explicit_period=off  period=1  equ=P=C  opselect=C  inp2=PCIN>>17  opr=+  inp1=P  carry=CIN  dbl_ovrd=off  block_type=constant
  Constant3 : xbsIndex_r4/Constant  const=-max_unwrap_periods  gui_display_data_type=Fixed-point  arith_type=Signed (2's comp)  n_bits=7  bin_pt=0  preci_type=Single  exp_width=8  frac_width=24  explicit_period=off  period=1  equ=P=C  opselect=C  inp2=PCIN>>17  opr=+  inp1=P  carry=CIN  dbl_ovrd=off  block_type=constant
  Constant4 : xbsIndex_r4/Constant  const=0  gui_display_data_type=Fixed-point  arith_type=Signed (2's comp)  n_bits=17  bin_pt=0  preci_type=Single  exp_width=8  frac_width=24  explicit_period=off  period=1  equ=P=C  opselect=C  inp2=PCIN>>17  opr=+  inp1=P  carry=CIN  dbl_ovrd=off  block_type=constant
  Constant5 : xbsIndex_r4/Constant  const=TDC_cnt_per_period  gui_display_data_type=Fixed-point  arith_type=Signed (2's comp)  n_bits=17  bin_pt=0  preci_type=Single  exp_width=8  frac_width=24  explicit_period=off  period=1  equ=P=C  opselect=C  inp2=PCIN>>17  opr=+  inp1=P  carry=CIN  dbl_ovrd=off  block_type=constant
  Constant6 : xbsIndex_r4/Constant  Commented=on  const=unwrap_res_thr  gui_display_data_type=Fixed-point  arith_type=Signed (2's comp)  n_bits=17  bin_pt=0  preci_type=Single  exp_width=8  frac_width=24  explicit_period=off  period=1  equ=P=C  opselect=C  inp2=PCIN>>17  opr=+  inp1=P  carry=CIN  dbl_ovrd=off  block_type=constant
  Constant7 : xbsIndex_r4/Constant  const=unwrap_res_period_thr  gui_display_data_type=Fixed-point  arith_type=Signed (2's comp)  n_bits=17  bin_pt=0  preci_type=Single  exp_width=8  frac_width=24  explicit_period=off  period=1  equ=P=C  opselect=C  inp2=PCIN>>17  opr=+  inp1=P  carry=CIN  dbl_ovrd=off  block_type=constant
  Constant8 : xbsIndex_r4/Constant  const=0  gui_display_data_type=Fixed-point  arith_type=Signed (2's comp)  n_bits=7  bin_pt=0  preci_type=Single  exp_width=8  frac_width=24  explicit_period=off  period=1  equ=P=C  opselect=C  inp2=PCIN>>17  opr=+  inp1=P  carry=CIN  dbl_ovrd=off  block_type=constant
  Constant9 : xbsIndex_r4/Constant  const=wrap_detect_thr+TDC_cnt_per_period  gui_display_data_type=Fixed-point  arith_type=Signed (2's comp)  n_bits=17  bin_pt=0  preci_type=Single  exp_width=8  frac_width=24  explicit_period=off  period=1  equ=P=C  opselect=C  inp2=PCIN>>17  opr=+  inp1=P  carry=CIN  dbl_ovrd=off  block_type=constant
  Delay : xbsIndex_r4/Delay  rst=off  infoeditControl=Selection of Reset will increase slice count due to use of real FFs and instead of SRLs  en=off  latency=1  reg_retiming=off  dbl_ovrd=off  block_type=delay
  Delay1 : xbsIndex_r4/Delay  rst=off  infoeditControl=Selection of Reset will increase slice count due to use of real FFs and instead of SRLs  en=off  latency=1  reg_retiming=off  dbl_ovrd=off  block_type=delay
  Logical1 : xbsIndex_r4/Logical  logical_function=AND  inputs=2  en=off  latency=0  precision=Full  arith_type=Unsigned  n_bits=16  bin_pt=0  align_bp=on  dbl_ovrd=off  block_type=logical
  Logical10 : xbsIndex_r4/Logical  logical_function=AND  inputs=2  en=off  latency=0  precision=Full  arith_type=Unsigned  n_bits=16  bin_pt=0  align_bp=on  dbl_ovrd=off  block_type=logical
  Logical9 : xbsIndex_r4/Logical  logical_function=AND  inputs=2  en=off  latency=0  precision=Full  arith_type=Unsigned  n_bits=16  bin_pt=0  align_bp=on  dbl_ovrd=off  block_type=logical
  Mult : xbsIndex_r4/Mult  precision=User Defined  arith_type="Signed  (2's comp)"  n_bits=17  bin_pt=0  quantization=Truncate  overflow=Saturate  en=off  latency=0  use_behavioral_HDL=off  opt=Speed  use_embedded=on  optimum_pipeline=off  pipeline=on  dbl_ovrd=off  use_rpm=on  placement_style=Triangular  block_type=mult
  Mux{1..7} (7 alike) : xbsIndex_r4/Mux  inputs=2  en=off  latency=0  precision=Full  arith_type=Unsigned  n_bits=16  bin_pt=14  quantization=Truncate  overflow=Wrap  dbl_ovrd=off  block_type=mux
  Register : xbsIndex_r4/Register  init=0  rst=on  en=off  dbl_ovrd=off  block_type=register
  Relational{,1,5..6} (4 alike) : xbsIndex_r4/Relational  mode=a>=b  op_type=Bool  en=off  latency=0  dbl_ovrd=off  block_type=relational
  Relational2 : xbsIndex_r4/Relational  mode=a<=b  op_type=Bool  en=off  latency=0  dbl_ovrd=off  block_type=relational
  Relational3 : xbsIndex_r4/Relational  mode=a<b  op_type=Bool  en=off  latency=0  dbl_ovrd=off  block_type=relational
  Relational4 : xbsIndex_r4/Relational  mode=a>b  op_type=Bool  en=off  latency=0  dbl_ovrd=off  block_type=relational
  num_correction_periods : xbsIndex_r4/Register  init=0  rst=on  en=off  dbl_ovrd=off  block_type=register
  sign : xbsIndex_r4/Slice  nbits=1  boolean_output=on  mode=Upper Bit Location + Width  bit1=0  base1=MSB of Input  bit0=0  base0=LSB of Input  dbl_ovrd=off  block_type=slice
  filt_reset : Outport
  unwr_cnts : Outport  Port=2
  wires:
  Logical10/1 -> Delay1/1, Mux6/1
  Constant2/1 -> Relational1/2, Mux3/3
  sign/1 -> Mux2/1
  AddSub2/1 -> Mux4/2, Relational2/1
  Delay/1 -> AddSub3/2, AddSub/1
  Relational4/1 -> Logical9/1
  num_correction_periods/1 -> AddSub1/1, Absolute2/1, AddSub2/1, Mux1/2
  AddSub1/1 -> Mux3/2, Relational1/1
  reset/1 -> num_correction_periods/2, Register/2
  Constant/1 -> Relational/2
  Relational2/1 -> Mux4/1
  Mult/1 -> Mux5/3
  Relational/1 -> Mux1/1
  AddSub/1 -> sign/1, Absolute/1
  freq_corr_feedback/1 -> Relational5/2, Relational3/1
  Mux2/1 -> Mux1/3
  Mux4/1 -> Mux2/3
  AddSub3/1 -> unwr_cnts/1
  Constant4/1 -> Mux5/2
  Logical9/1 -> Logical10/1
  Mux3/1 -> Mux2/2
  Absolute/1 -> Relational6/1, Relational/1
  Relational1/1 -> Mux3/1
  Mux5/1 -> AddSub3/1
  Constant3/1 -> Relational2/2, Mux4/3
  DT_cnts/1 -> AddSub4/1
  Mux6/1 -> Mult/1, num_correction_periods/1
  Constant8/1 -> Mux6/3
  Constant7/1 -> Relational4/2
  Absolute2/1 -> Relational4/1
  Constant5/1 -> Mult/2
  Mux1/1 -> Mux6/2
  unwr_en/1 -> Mux5/1
  reset_enable/1 -> Logical10/2
  Delay1/1 -> filt_reset/1
  setpoint_cnts/1 -> Register/1
  unwr_res_thr/1 -> Relational3/2
  prev_freq_corr_feedback/1 -> Relational5/1
  Relational5/1 -> Logical1/1
  Relational3/1 -> Logical1/2
  Logical1/1 -> Logical9/2
  Constant9/1 -> Relational6/2
  Relational6/1 -> Mux7/1
  Mux7/1 -> AddSub2/2, AddSub1/2
  Constant1/1 -> Mux7/2
  Constant10/1 -> Mux7/3
  AddSub4/1 -> AddSub/2, Delay/1
  Register/1 -> AddSub4/2
